simulink library "discreteSecondOrderPD_cl"  (R2022a)
settings: Solver=VariableStepAuto  StartTime=0.0  StopTime=10.0  RelTol=1e-3
undefined symbols (not defined in the file): Ts
libraries: discreteFilter_ul x2
settings Model: Creator=adabney  LastModifiedBy=adabney

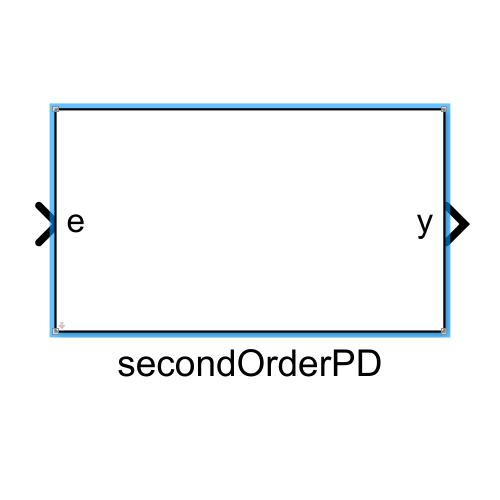
[thumbnail: Simulink's stored preview of the top-level diagram]
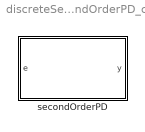
== system discreteSecondOrderPD_cl ==
  secondOrderPD : Subsystem  mask{kP=0, kD=0, tauReference=0, tauDerivative=0, Ts=Ts}
      mask prompts: kP "Proportional Gain"; kD "Derivative Gain"; tauReference "Reference Filter Time Constant"; tauDerivative "Derivative Filter Time Constant"; Ts "Sample Time"
      mask DialogControl DescTextVar Prompt: Mask for inputting controller gains for a second order filtered PD controller
      mask DialogControl ParameterGroupVar Prompt: Gains

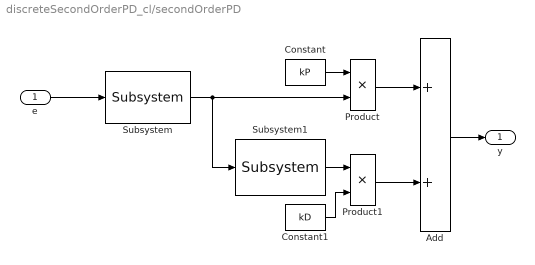
== system discreteSecondOrderPD_cl/secondOrderPD ==
  e : Inport
  Add : Sum
  Constant : Constant  Value=kP
  Constant1 : Constant  Value=kD
  Product : Product
  Product1 : Product
  Subsystem : discreteFilter_ul/Subsystem  Ts=Ts  tau=tauReference
  Subsystem1 : discreteFilter_ul/Subsystem  Ts=Ts  tau=tauDerivative
  y : Outport
  wires:
  e/1 -> Subsystem/1
  Subsystem/1 -> Product/2, Subsystem1/1
  Subsystem1/1 -> Product1/1
  Add/1 -> y/1
  Product/1 -> Add/1
  Product1/1 -> Add/2
  Constant1/1 -> Product1/2
  Constant/1 -> Product/1
